simulink model "lab3a"  (R2022b)
settings: Solver=FixedStepAuto  StartTime=0.0  StopTime=1.0  FixedStep=1/1024  RelTol=1e-3
values from neighbouring files (symbols this model uses):
  i = 2^b    [lab3a_script.m]
undefined symbols (not defined in the file or in its folder): lutdata, lutix
settings Model: Creator=simja  LastModifiedBy=simja
settings DataIOCC: ReturnWorkspaceOutputs=off

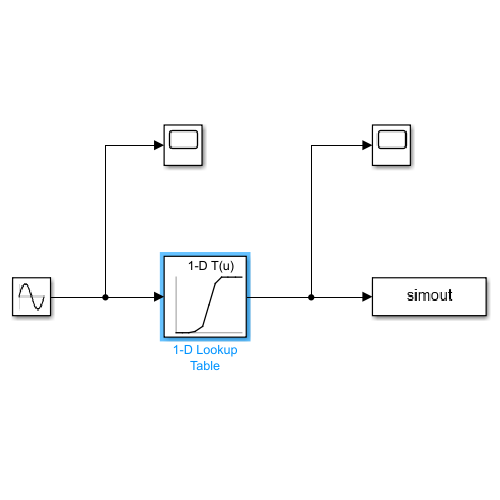
[thumbnail: Simulink's stored preview of the top-level diagram]
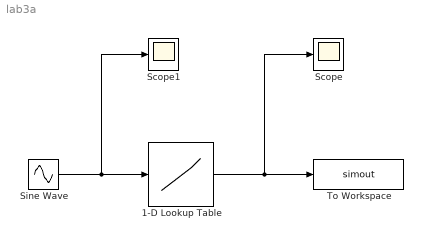
== system lab3a ==
  1-D Lookup Table : Lookup_n-D  NumberOfTableDimensions=1  BreakpointsForDimension1=lutix(i)  Table=lutdata(i)  InternalRulePriority=Speed  RndMeth=Simplest
  Scope : Scope
  Scope1 : Scope
  Sine Wave : Sin  Frequency=2*5*pi  SampleTime=0
  To Workspace : ToWorkspace  VariableName=simout  SaveFormat=Structure With Time  SampleTime=-1
  wires:
  Sine Wave/1 -> Scope1/1, 1-D Lookup Table/1
  1-D Lookup Table/1 -> Scope/1, To Workspace/1
